simulink model "sim_motor"  (R2025b)
settings: Solver=FixedStepAuto  StartTime=0.0  StopTime=inf  FixedStep=0.02  MaxStep=0.02  RelTol=1e-3  AbsTol=1e-3
undefined symbols (not defined in the file or in its folder): f, rad, s
libraries: nesl_utility x6, fl_lib x4, ee_lib x3, instrumentlib x2, aerolibconvert2 x1, mcbplantlib x1, simulink x1
settings Model: Creator=Francisco  LastModifiedBy=Francisco
settings SolverCC: AutoScaleAbsTol=off  AlgebraicLoopSolver=TrustRegion  MaxZcPerStep=1.0
settings DebuggingCC: UnconnectedInputMsg=warning  UnconnectedOutputMsg=warning  UnconnectedLineMsg=warning  SymbolicDimsDataTypeCodeGenerationDiagnostic=none
settings ModelReferenceCC: EnableRefExpFcnMdlSchedulingChecks=on
settings SFSimCC: CustomCodeUndefinedFunction=UseInterfaceOnly
settings RTWCC: GPUComputeCapability=3.5  DLArmComputeVersion=19.05
settings SimscapeCC: SimscapeLogType=all  SimscapeLogSimulationStatistics=on  SimscapeLogDataHistory=10000.0

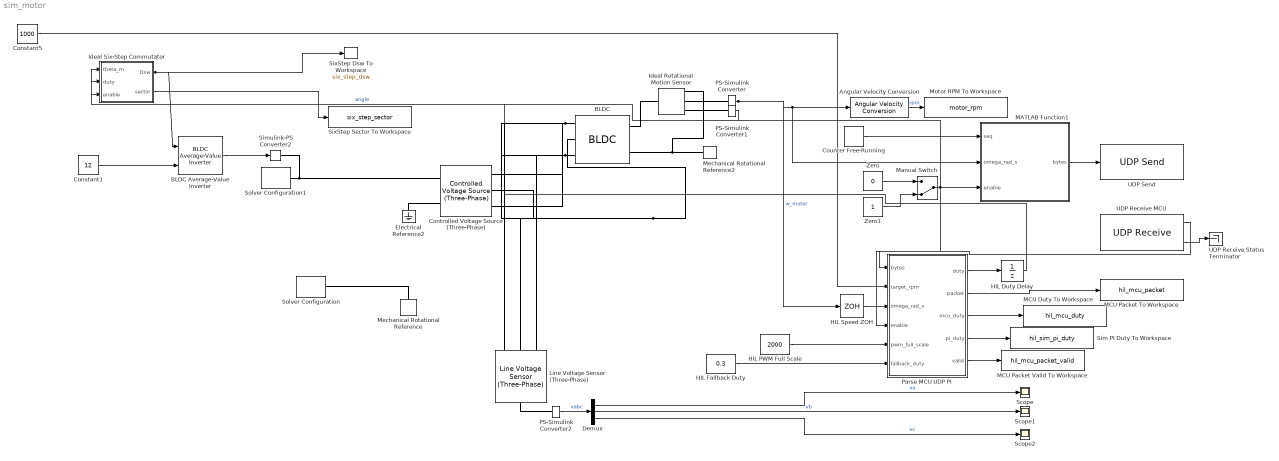
== system sim_motor ==
  Angular Velocity Conversion : aerolibconvert2/Angular Velocity Conversion  IU=rad/s  OU=rpm
  BLDC : ee_lib/Electromechanical/Permanent Magnet/BLDC  port_option=ee.enum.threePhasePort.expanded  rotor_param=ee.enum.pmsm.backemf.trapezoidbackemf  pm_flux_linkage=0.03 Wb  theta_constant=pi/12 rad  emf_max=0.5 V  w_meas=474.6 rpm  DphiDtheta_tab=[0, -.1528, -.1528, .1528, .1528, 0] Wb/rad  back_emf_tab=[0, -9.6, -9.6, 9.6, 9.6, 0] V  rotor_angle_tab=[0, 7.5, 22.5, 37.5, 52.5, 60] deg  nPolePairs=2  axes_param=ee.enum.rotorangle.daxis  winding_type=ee.enum.electromech.statorconfiguration.wye  stator_param=ee.enum.statorparam.LsLmMs  machine_param=ee.enum.dqparameterization.constant  Ld=0.00022 H  Lq=0.00022 H  idVec=[-200, 0, 200] A  iqVec=[-200, 0, 200] A  LdMatrix=0.00022 * ones(3, 3) H  LqMatrix=0.00022 * ones(3, 3) H  L0=0.00016 H  Ls=1.63 mH  Lm=0 H  Ms=0 H  Rs=2 Ohm  zero_sequence=ee.enum.park.zerosequence.exclude  loss_param=ee.enum.ironloss.none  losses_oc=[0, 0, 0] W  losses_sc=[0, 0, 0] W  f_losses=60 Hz  Isc_losses=95 A  J=72.9e-6 kg*m^2  lam=1e-5 N*m*s/rad  i_d_specify=on  i_d_priority=None  i_d=0 A  i_d_nominal_specify=off  i_d_nominal_value=1  i_d_nominal_unit=A  i_q_specify=on  i_q_priority=None  i_q=0 A  i_q_nominal_specify=off  i_q_nominal_value=1  i_q_nominal_unit=A  torque_specify=on  torque_priority=None  torque=0 N*m  torque_nominal_specify=off  torque_nominal_value=1  torque_nominal_unit=N*m  angular_velocity_specify=on  angular_velocity_priority=High  angular_velocity=0 rpm  angular_velocity_nominal_specify=off  angular_velocity_nominal_value=1  angular_velocity_nominal_unit=rpm  angular_position_specify=on  angular_position_priority=High  angular_position=0 deg  angular_position_nominal_specify=off  angular_position_nominal_value=1  angular_position_nominal_unit=deg  alpha=3.93e-3 1/K  alpha_flux=-0.001 1/K  Tmeas=298.15 K  stator_thermal_mass=100 J/K  rotor_thermal_mass=200 J/K  Rm_percent_rotor=90  Rd_percent_rotor=30  temperatureA_specify=off  temperatureA_priority=High  temperatureA=25 degC  temperatureA_nominal_specify=off  temperatureA_nominal_value=1  temperatureA_nominal_unit=degC  temperatureB_specify=off  temperatureB_priority=High  temperatureB=25 degC  temperatureB_nominal_specify=off  temperatureB_nominal_value=1  temperatureB_nominal_unit=degC  temperatureC_specify=off  temperatureC_priority=High  temperatureC=25 degC  temperatureC_nominal_specify=off  temperatureC_nominal_value=1  temperatureC_nominal_unit=degC  temperatureR_specify=off  temperatureR_priority=High  temperatureR=25 degC  temperatureR_nominal_specify=off  temperatureR_nominal_value=1  temperatureR_nominal_unit=degC
      settings: InternalSimscapePortConfiguration="{\"Bottom\":[],\"Left\":[{\"id\":\"a\",\"label\":\"a\",\"type\":\"foundation.electrical.electrical\"},{\"id\":\"b\",\"label\":\"b\",\"type\":\"foundation.electrical.electrical\"},{\"id\":\"c\",\"label\":\"c\",\"type\":\"foundation.electrical.electrical\"}],\"Right\":[{\"id\":\"R\",\"label\":\"R\",\"type\":\"foundation.mechanical.rotational.rotational\"},{\"id\":\"C\",\"label\":\"C\",\"type\":\"foundation.mechanical.rotational.rotational\"}],\"Top\":[]}"
  BLDC Average-Value Inverter : mcbplantlib/BLDC Average-Value Inverter
      settings: LibrarySourceBlock=mcblib/Electrical Systems/Inverters/BLDC Average-Value Inverter
  Constant1 : Constant  Value=12
  Constant5 : Constant  Value=1000
  Controlled Voltage Source (Three-Phase) : ee_lib/Sources/Controlled Voltage Source (Three-Phase)  input_option=ee.enum.inputType.instantaneous  FRated=60 Hz
      settings: InternalSimscapePortConfiguration="{\"Bottom\":[],\"Left\":[{\"id\":\"S\",\"label\":\"S\",\"type\":\"input\"},{\"id\":\"n\",\"label\":\"n\",\"type\":\"foundation.electrical.electrical\"}],\"Right\":[{\"id\":\"a\",\"label\":\"a\",\"type\":\"foundation.electrical.electrical\"},{\"id\":\"b\",\"label\":\"b\",\"type\":\"foundation.electrical.electrical\"},{\"id\":\"c\",\"label\":\"c\",\"type\":\"foundation.electrical.electrical\"}],\"Top\":[]}"
  Counter Free-Running : simulink/Sources/Counter Free-Running  NumBits=8  tsamp=0.02
  Demux : Demux  Outputs=3
  Electrical Reference2 : fl_lib/Electrical/Electrical Elements/Electrical Reference
  HIL Duty Delay : UnitDelay  InitialCondition=0.3  SampleTime=0.02  HasFrameUpgradeWarning=on
  HIL Fallback Duty : Constant  Value=0.3  SampleTime=0.02
  HIL PWM Full Scale : Constant  Value=2000  SampleTime=0.02
  HIL Speed ZOH : ZeroOrderHold  SampleTime=0.02
  Ideal Rotational Motion Sensor : fl_lib/Mechanical/Mechanical Sensors/Ideal Rotational Motion Sensor  reference=foundation.enum.MeasurementReference.difference  acceleration_port=false  velocity_port=true  position_port=true  wrap_angle=false  offset=0 rad
  Ideal Six-Step Commutator : MATLAB Function  TreatAsAtomicUnit=on  SystemSampleTime=1e-3
  Line Voltage Sensor (Three-Phase) : ee_lib/Sensors & Transducers/Line Voltage Sensor (Three-Phase)
      settings: InternalSimscapePortConfiguration="{\"Bottom\":[],\"Left\":[{\"id\":\"a\",\"label\":\"a\",\"type\":\"foundation.electrical.electrical\"},{\"id\":\"b\",\"label\":\"b\",\"type\":\"foundation.electrical.electrical\"},{\"id\":\"c\",\"label\":\"c\",\"type\":\"foundation.electrical.electrical\"}],\"Right\":[{\"id\":\"V_output\",\"label\":\"V\",\"type\":\"output\"}],\"Top\":[]}"
  MATLAB Function1 : MATLAB Function  TreatAsAtomicUnit=on
  MCU Duty To Workspace : ToWorkspace  VariableName=hil_mcu_duty  SampleTime=-1
      settings: MaxDataPoints=5000
  MCU Packet To Workspace : ToWorkspace  VariableName=hil_mcu_packet  SampleTime=-1
      settings: MaxDataPoints=5000
  MCU Packet Valid To Workspace : ToWorkspace  VariableName=hil_mcu_packet_valid  SampleTime=-1
      settings: MaxDataPoints=5000
  Manual Switch : ManualSwitch  CurrentSetting=0
  Mechanical Rotational Reference : fl_lib/Mechanical/Rotational Elements/Mechanical Rotational Reference
  Mechanical Rotational Reference2 : fl_lib/Mechanical/Rotational Elements/Mechanical Rotational Reference
  Motor RPM To Workspace : ToWorkspace  VariableName=motor_rpm  SampleTime=-1
      settings: MaxDataPoints=5000
  PS-Simulink Converter : nesl_utility/PS-Simulink Converter  PhysicalDomain=network_engine_domain  SubClassName=ps_output  LeftPortType=input  RightPortType=output  PseudoPeriodic=off  Frequencies=[]  VectorFormat=inherit  Unit=inherit  AffineConversion=off
  PS-Simulink Converter1 : nesl_utility/PS-Simulink Converter  PhysicalDomain=network_engine_domain  SubClassName=ps_output  LeftPortType=input  RightPortType=output  PseudoPeriodic=off  Frequencies=[]  VectorFormat=inherit  Unit=rad  AffineConversion=off
  PS-Simulink Converter2 : nesl_utility/PS-Simulink Converter  PhysicalDomain=network_engine_domain  SubClassName=ps_output  LeftPortType=input  RightPortType=output  PseudoPeriodic=off  Frequencies=[]  VectorFormat=inherit  Unit=inherit  AffineConversion=off
  Parse MCU UDP PI : MATLAB Function  TreatAsAtomicUnit=on  SystemSampleTime=0.02
  Scope : Scope
      settings: ActiveDisplayYMinimum=-9.0978113857563816  ActiveDisplayYMaximum=8.4733530232311143
  Scope1 : Scope
  Scope2 : Scope
      settings: DataLoggingVariableName=ScopeData2
  Sim PI Duty To Workspace : ToWorkspace  VariableName=hil_sim_pi_duty  SampleTime=-1
      settings: MaxDataPoints=5000
  Simulink-PS Converter2 : nesl_utility/Simulink-PS Converter  PhysicalDomain=network_engine_domain  SubClassName=ps_input  LeftPortType=input  RightPortType=output  PseudoPeriodic=off  Frequencies=[]  NoiseDistribution=none  NoiseParameters=[]  Unit=V  AffineConversion=off  FilteringAndDerivatives=provide  SimscapeFilterOrder=1  InputFilterTimeConstant=0.001  UdotUserProvided=0
  SixStep Dsw To Workspace : ToWorkspace  VariableName=six_step_dsw  SampleTime=-1
      settings: MaxDataPoints=5000
  SixStep Sector To Workspace : ToWorkspace  VariableName=six_step_sector  SampleTime=-1
      settings: MaxDataPoints=5000
  Solver Configuration : nesl_utility/Solver Configuration  PhysicalDomain=network_engine_domain  SubClassName=solver  LeftPortType=input  RightPortType=generic  Tones=[]  Harmonics=[]  SimulateNoise=off  Profile=off  UseLocalSampling=off  EnableSwitchedLinearOptims=on  FrequencyDomain=off  UseCCode=off  RelTol=0.001  AbsTol=1e-06  MinStep=1e-09  ToWorkspace=off  RevertToSquareIcSolve=off  NumHomotopyIterations=100  PhasorMode=off  PhasorModeNumHarmonics=1  ConsistencySolver=NEWTON_XTOL_AFTER_FTOL  IndexReductionMethod=DerivativeReplacement  DoDC=off  ResidualTolerance=1e-09  ConsistencyTolSource=GLOBAL  ConsistencyAbsTol=0.001  ConsistencyRelTol=0.001  ConsistencyTolFactor=0.001  UseLocalSolver=off  LocalSolverChoice=NE_BACKWARD_EULER_ADVANCER  ResolveIndetEquations=on  FunctionEvalNumThread=1  LocalSolverSampleTime=0.001  DoFixedCost=off  MaxNonlinIter=3  MaxModeIter=2  ComputeImpulses=off  ImpulseIterations=2  LinearAlgebra=auto  LinearAlgebraNumThread=0  EquationFormulation=NE_TIME_EF  DelaysMemoryBudget=1024  AutomaticFiltering=on  FilteringTimeConstant=0.001  PartitionStorageMethod=AS_NEEDED  PartitionMemoryBudget=1024  PartitionMethod=ROBUST  MultibodyUseLocalSolver=off  MultibodyLocalSolverChoice=ODE1  MultibodyLocalSolverSampleTime=0.001
  Solver Configuration1 : nesl_utility/Solver Configuration  PhysicalDomain=network_engine_domain  SubClassName=solver  LeftPortType=input  RightPortType=generic  Tones=[]  Harmonics=[]  SimulateNoise=off  Profile=off  UseLocalSampling=off  EnableSwitchedLinearOptims=on  FrequencyDomain=off  UseCCode=off  RelTol=0.001  AbsTol=1e-06  MinStep=1e-09  ToWorkspace=off  RevertToSquareIcSolve=off  NumHomotopyIterations=100  PhasorMode=off  PhasorModeNumHarmonics=1  ConsistencySolver=NEWTON_XTOL_AFTER_FTOL  IndexReductionMethod=DerivativeReplacement  DoDC=off  ResidualTolerance=1e-09  ConsistencyTolSource=GLOBAL  ConsistencyAbsTol=0.001  ConsistencyRelTol=0.001  ConsistencyTolFactor=0.001  UseLocalSolver=off  LocalSolverChoice=NE_BACKWARD_EULER_ADVANCER  ResolveIndetEquations=on  FunctionEvalNumThread=1  LocalSolverSampleTime=0.001  DoFixedCost=off  MaxNonlinIter=3  MaxModeIter=2  ComputeImpulses=off  ImpulseIterations=2  LinearAlgebra=auto  LinearAlgebraNumThread=0  EquationFormulation=NE_TIME_EF  DelaysMemoryBudget=1024  AutomaticFiltering=on  FilteringTimeConstant=0.001  PartitionStorageMethod=AS_NEEDED  PartitionMemoryBudget=1024  PartitionMethod=ROBUST  MultibodyUseLocalSolver=off  MultibodyLocalSolverChoice=ODE1  MultibodyLocalSolverSampleTime=0.001
  UDP Receive MCU : instrumentlib/UDP Receive  LocalAddress=0.0.0.0  LocalPort=5058  EnablePortSharing=on  Host=127.0.0.1  Port=5057  GetLatestData=on  DataSize=[1, 256]  DataType=uint8  ASCIIFormatting=%f,  Terminator=LF  CustomTerminator=10  ByteOrder=big-endian  EnableBlockingMode=off  Timeout=0.001  SampleTime=0.01  SimulateUsing=Interpreted execution
  UDP Receive Status Terminator : Terminator
  UDP Send : instrumentlib/UDP Send  Host=127.0.0.1  Port=5057  LocalAddress=0.0.0.0  LocalPort=5058  EnablePortSharing=on  OutputDatagramPacketSize=64  ByteOrder=big-endian  EnableBlockingMode=off  SimulateUsing=Interpreted execution
  Zero : Constant  Value=0  OutDataTypeStr=Inherit: Inherit via back propagation
  Zero1 : Constant  OutDataTypeStr=Inherit: Inherit via back propagation
  wires:
  BLDC Average-Value Inverter/1 -> Simulink-PS Converter2/1
  Constant1/1 -> BLDC Average-Value Inverter/2
  Ideal Six-Step Commutator/1(Dsw) -> BLDC Average-Value Inverter/1, SixStep Dsw To Workspace/1
  PS-Simulink Converter/1 -> MATLAB Function1/2(omega_rad_s), Angular Velocity Conversion/1, HIL Speed ZOH/1  "w_motor"
  PS-Simulink Converter2/1 -> Demux/1  "vabc"
  Demux/1 -> Scope/1  "va"
  Demux/2 -> Scope1/1  "vb"
  Demux/3 -> Scope2/1  "vc"
  MATLAB Function1/1(bytes) -> UDP Send/1
  Counter Free-Running/1 -> MATLAB Function1/1(seq)
  Zero/1 -> Manual Switch/1
  Zero1/1 -> Manual Switch/2
  Manual Switch/1 -> MATLAB Function1/3(enable), Parse MCU UDP PI/4(enable), Ideal Six-Step Commutator/3(enable)
  UDP Receive MCU/1 -> Parse MCU UDP PI/1(bytes)
  UDP Receive MCU/2 -> UDP Receive Status Terminator/1
  Constant5/1 -> Parse MCU UDP PI/2(target_rpm)
  HIL Speed ZOH/1 -> Parse MCU UDP PI/3(omega_rad_s)
  HIL PWM Full Scale/1 -> Parse MCU UDP PI/5(pwm_full_scale)
  HIL Fallback Duty/1 -> Parse MCU UDP PI/6(fallback_duty)
  Parse MCU UDP PI/1(duty) -> HIL Duty Delay/1
  Parse MCU UDP PI/2(packet) -> MCU Packet To Workspace/1
  Parse MCU UDP PI/3(mcu_duty) -> MCU Duty To Workspace/1
  Parse MCU UDP PI/4(pi_duty) -> Sim PI Duty To Workspace/1
  Parse MCU UDP PI/5(valid) -> MCU Packet Valid To Workspace/1
  Angular Velocity Conversion/1 -> Motor RPM To Workspace/1  "rpm"
  PS-Simulink Converter1/1 -> Ideal Six-Step Commutator/1(theta_m)  "angle"
  HIL Duty Delay/1 -> Ideal Six-Step Commutator/2(duty)
  Ideal Six-Step Commutator/2(sector) -> SixStep Sector To Workspace/1
  connections:
  Solver Configuration/RConn1 -- Mechanical Rotational Reference/LConn1
  Mechanical Rotational Reference2/LConn1 -- BLDC/RConn2 -- Ideal Rotational Motion Sensor/RConn1
  Solver Configuration1/RConn1 -- Simulink-PS Converter2/RConn1 -- Controlled Voltage Source (Three-Phase)/LConn1
  Controlled Voltage Source (Three-Phase)/LConn2 -- Electrical Reference2/LConn1
  BLDC/RConn1 -- Ideal Rotational Motion Sensor/LConn1
  Ideal Rotational Motion Sensor/RConn2 -- PS-Simulink Converter/LConn1
  Ideal Rotational Motion Sensor/RConn3 -- PS-Simulink Converter1/LConn1
  Line Voltage Sensor (Three-Phase)/RConn1 -- PS-Simulink Converter2/LConn1
  Controlled Voltage Source (Three-Phase)/RConn2 -- BLDC/LConn2 -- Line Voltage Sensor (Three-Phase)/LConn2
  BLDC/LConn1 -- Controlled Voltage Source (Three-Phase)/RConn1 -- Line Voltage Sensor (Three-Phase)/LConn1
  BLDC/LConn3 -- Controlled Voltage Source (Three-Phase)/RConn3 -- Line Voltage Sensor (Three-Phase)/LConn3

== matlab function sim_motor/MATLAB Function1 ==
  data: seq input; bytes output uint8 size=[1 32]; omega_rad_s input; enable input
function bytes = build_pil_packet(seq, omega_rad_s, enable)
%#codegen

bytes = zeros(1, 32, 'uint8');   % salida fija

rpm = round(omega_rad_s * 60 / (2*pi));
rpm = max(0, min(65535, rpm));

seq_u32 = uint32(seq);
rpm_u16 = uint16(rpm);
en_u8   = uint8(enable ~= 0);

msg = uint8(sprintf('%u,%u,%u', seq_u32, rpm_u16, en_u8));

n = min(numel(msg), numel(bytes));
bytes(1:n) = msg(1:n);
end

== matlab function sim_motor/Ideal Six-Step Commutator ==
  data: theta_m input; Dsw output; duty input; enable input; sector output
function [Dsw, sector] = ideal_six_step_commutator(theta_m, duty, enable)
%#codegen

% BLDC block has two pole pairs. theta_m arrives in radians.
pole_pairs = 2.0;
electrical_offset = 0.0;
Dsw = zeros(1, 6);
sector = 0.0;

if enable == 0
    return;
end

d = min(1.0, max(0.0, double(duty)));
theta_e = mod(pole_pairs * double(theta_m) + electrical_offset, 2.0*pi);
sector = floor(theta_e / (2.0*pi/6.0)) + 1.0;
if sector > 6.0
    sector = 6.0;
end

switch sector
    case 1
        Dsw = [d 0 0 0 0 1]; % A+ C-
    case 2
        Dsw = [d 0 0 1 0 0]; % A+ B-
    case 3
        Dsw = [0 0 0 1 d 0]; % C+ B-
    case 4
        Dsw = [0 1 0 0 d 0]; % C+ A-
    case 5
        Dsw = [0 1 d 0 0 0]; % B+ A-
    otherwise
        Dsw = [0 0 d 0 0 1]; % B+ C-
end

== matlab function sim_motor/Parse MCU UDP PI ==
  data: bytes input; duty output; target_rpm input; omega_rad_s input; enable input; pwm_full_scale input; fallback_duty input; packet output; mcu_duty output; pi_duty output; valid output
function [duty, packet, mcu_duty, pi_duty, valid] = hil_udp_packet_pi(bytes, target_rpm, omega_rad_s, enable, pwm_full_scale, fallback_duty)
%#codegen

persistent integral
if isempty(integral)
    integral = 0.0;
end

packet = zeros(1, 16);
numbers = zeros(1, 15);
valid = false;
mcu_duty = 0.0;
full_scale = max(1.0, double(pwm_full_scale));
fallback = min(1.0, max(0.0, double(fallback_duty)));

% Local PI reference in duty units. It is logged, not used as the
% plant command unless the MCU packet path is made valid upstream.
Ts = 0.02;
Kp = 6.0e-4;
Ki = 2.0e-4;
rpm_meas = omega_rad_s * 60.0 / (2.0*pi);
err = target_rpm - rpm_meas;
if enable == 0
    integral = 0.0;
end
u = Kp * err + integral;
pi_duty = min(1.0, max(0.0, u));
if (u > 0.0 && u < 1.0) || (u <= 0.0 && err > 0.0) || (u >= 1.0 && err < 0.0)
    integral = integral + Ki * err * Ts;
end
pi_duty = min(1.0, max(0.0, Kp * err + integral));

raw = uint8(bytes(:));
n = numel(raw);
start = 1;
% UDP Receive prepends the datagram length to uint8 payloads.
if n >= 5 && raw(1) ~= 111 && raw(1) ~= 79 && ...
        (raw(2) == 111 || raw(2) == 79) && ...
        (raw(3) == 107 || raw(3) == 75) && raw(4) == 44
    start = 2;
end
if n - start + 1 >= 4
    is_ok = (raw(start) == 111 || raw(start) == 79) && ... % o/O
            (raw(start + 1) == 107 || raw(start + 1) == 75) && ... % k/K
            raw(start + 2) == 44;
    if is_ok
        index = 1;
        value = 0.0;
        sign_value = 1.0;
        fraction = 0.1;
        in_fraction = false;
        have_digit = false;
        for k = start + 3:n
            c = raw(k);
            if c == 0 || c == 10 || c == 13
                break;
            elseif c == 44
                if have_digit && index <= 15
                    numbers(index) = sign_value * value;
                    index = index + 1;
                end
                value = 0.0;
                sign_value = 1.0;
                fraction = 0.1;
                in_fraction = false;
                have_digit = false;
            elseif c == 45
                sign_value = -1.0;
            elseif c == 46
                in_fraction = true;
            elseif c >= 48 && c <= 57
                have_digit = true;
                digit = double(c - 48);
                if in_fraction
                    value = value + digit * fraction;
                    fraction = fraction * 0.1;
                else
                    value = value * 10.0 + digit;
                end
            end
        end
        if have_digit && index <= 15
            numbers(index) = sign_value * value;
            index = index + 1;
        end
        valid = index > 15;
    end
end

if valid
    packet(1) = 1.0;
    for k = 1:15
        packet(k + 1) = numbers(k);
    end
    mcu_duty = min(1.0, max(0.0, numbers(7) / full_scale));
end

if enable ~= 0
    if valid
        duty = mcu_duty;
    else
        duty = fallback;
    end
else
    duty = 0.0;
end
end
